simulink model "kalman_estimate_MM"  (R2018b)
settings: Solver=FixedStepAuto  StartTime=0.0  StopTime=500  FixedStep=0.02  RelTol=1e-3
values from neighbouring files (symbols this model uses):
  D = randn(num_output,num_control)    [Com_of_linear_model_calculate.m]    (also in Copy_of_linear_model_calculate.m; D.mat = [0 0 0.00507528406191 0.0236369284061 0.221173094143 0.00198; LINEAR.m = randn(8,1)*10; MM_HKF.m = reshape(out(A_l+B_l+C_l+1:A_l+B_l+C_l+D_l),size_D))
undefined symbols (not defined in the file or in its folder): act_piece, com_piece, piece, sigbuilder_block
libraries: sharedschedule x467, dspsigattribs x44, commchan3 x1
(part 5 of 5)

== system kalman_estimate_MM/sen2_PIECE kalman2/kalman filter1 ==
  A : Inport
  B : Inport  Port=2
  C : Inport  Port=3
  D : Inport  Port=4
  K : Inport  Port=5
  x0 : Inport  Port=6
  Y : Inport  Port=7
  U : Inport  Port=8
  Xtrim : Inport  Port=9
  "\tCX" : Product  Multiplication=Matrix(*)
  AX : Product  Multiplication=Matrix(*)
  BU : Product  Multiplication=Matrix(*)
  Convert 1-D to 2-D1 : dspsigattribs/Convert 1-D to 2-D  M=2  N=1  frameBasedOut=off
      settings: SourceProductName=DSP System Toolbox  SourceProductBaseCode=DS
  DU : Product  Multiplication=Matrix(*)
  Delay : Delay  DelayLength=1  InitialConditionSource=Input port
      settings: InputPortMap=u0,p4
  KY : Product  Multiplication=Matrix(*)
  MATLAB Function : MATLAB Function  TreatAsAtomicUnit=on
  Minus : Sum  Inputs=+-
  Minus1 : Sum
  Minus2 : Sum  Inputs=+-
  Minus3 : Sum  Inputs=+++
  Minus4 : Sum
  X_es : Outport
  Y_es : Outport  Port=2
  Y_error : Outport  Port=3
  wires:
  MATLAB Function/1(y) -> KY/2, Y_error/1
  Minus2/1 -> MATLAB Function/1(u)
  Convert 1-D to 2-D1/1 -> Delay/2
  x0/1 -> Convert 1-D to 2-D1/1
  Minus4/1 -> Minus2/2, Y_es/1
  KY/1 -> Minus3/1
  U/1 -> BU/2, DU/2
  Y/1 -> Minus2/1
  DU/1 -> Minus4/2
  "\tCX"/1 -> Minus4/1
  BU/1 -> Minus3/3
  A/1 -> AX/1
  B/1 -> BU/1
  C/1 -> "\tCX"/1
  D/1 -> DU/1
  K/1 -> KY/1
  Xtrim/1 -> Minus1/2, Minus/2
  Delay/1 -> Minus/1, X_es/1
  Minus/1 -> AX/2, "\tCX"/2
  AX/1 -> Minus3/2
  Minus3/1 -> Minus1/1
  Minus1/1 -> Delay/1

== system kalman_estimate_MM/sen2_PWL/kalman filter1 ==
  A : Inport
  B : Inport  Port=2
  C : Inport  Port=3
  D : Inport  Port=4
  x0 : Inport  Port=5
  U : Inport  Port=6
  Xtrim : Inport  Port=7
  "\tCX" : Product  Multiplication=Matrix(*)
  AX : Product  Multiplication=Matrix(*)
  BU : Product  Multiplication=Matrix(*)
  Convert 1-D to 2-D1 : dspsigattribs/Convert 1-D to 2-D  M=2  N=1  frameBasedOut=off
      settings: SourceProductName=DSP System Toolbox  SourceProductBaseCode=DS
  DU : Product  Multiplication=Matrix(*)
  Delay : Delay  DelayLength=1  InitialConditionSource=Input port
      settings: InputPortMap=u0,p4
  Minus : Sum  Inputs=+-
  Minus1 : Sum
  Minus3 : Sum
  Minus4 : Sum
  X_es : Outport
  Y_es : Outport  Port=2
  wires:
  BU/1 -> Minus3/1
  Convert 1-D to 2-D1/1 -> Delay/2
  x0/1 -> Convert 1-D to 2-D1/1
  Minus4/1 -> Y_es/1
  U/1 -> BU/2, DU/2
  DU/1 -> Minus4/2
  "\tCX"/1 -> Minus4/1
  A/1 -> AX/1
  B/1 -> BU/1
  C/1 -> "\tCX"/1
  D/1 -> DU/1
  Xtrim/1 -> Minus1/2, Minus/2
  Delay/1 -> Minus/1, X_es/1
  Minus/1 -> AX/2, "\tCX"/2
  AX/1 -> Minus3/2
  Minus3/1 -> Minus1/1
  Minus1/1 -> Delay/1

== system kalman_estimate_MM/sen3_PIECE kalman1/kalman filter1 ==
  A : Inport
  B : Inport  Port=2
  C : Inport  Port=3
  D : Inport  Port=4
  K : Inport  Port=5
  x0 : Inport  Port=6
  Y : Inport  Port=7
  U : Inport  Port=8
  Xtrim : Inport  Port=9
  "\tCX" : Product  Multiplication=Matrix(*)
  AX : Product  Multiplication=Matrix(*)
  BU : Product  Multiplication=Matrix(*)
  Convert 1-D to 2-D1 : dspsigattribs/Convert 1-D to 2-D  M=2  N=1  frameBasedOut=off
      settings: SourceProductName=DSP System Toolbox  SourceProductBaseCode=DS
  DU : Product  Multiplication=Matrix(*)
  Delay : Delay  DelayLength=1  InitialConditionSource=Input port
      settings: InputPortMap=u0,p4
  KY : Product  Multiplication=Matrix(*)
  MATLAB Function : MATLAB Function  TreatAsAtomicUnit=on
  Minus : Sum  Inputs=+-
  Minus1 : Sum
  Minus2 : Sum  Inputs=+-
  Minus3 : Sum  Inputs=+++
  Minus4 : Sum
  X_es : Outport
  Y_es : Outport  Port=2
  Y_error : Outport  Port=3
  wires:
  Minus1/1 -> Delay/1
  Minus3/1 -> Minus1/1
  AX/1 -> Minus3/2
  Minus/1 -> "\tCX"/2, AX/2
  Delay/1 -> X_es/1, Minus/1
  Xtrim/1 -> Minus/2, Minus1/2
  K/1 -> KY/1
  D/1 -> DU/1
  C/1 -> "\tCX"/1
  B/1 -> BU/1
  A/1 -> AX/1
  BU/1 -> Minus3/3
  "\tCX"/1 -> Minus4/1
  DU/1 -> Minus4/2
  Y/1 -> Minus2/1
  U/1 -> DU/2, BU/2
  KY/1 -> Minus3/1
  Minus4/1 -> Y_es/1, Minus2/2
  x0/1 -> Convert 1-D to 2-D1/1
  Convert 1-D to 2-D1/1 -> Delay/2
  Minus2/1 -> MATLAB Function/1(u)
  MATLAB Function/1(y) -> Y_error/1, KY/2

== system kalman_estimate_MM/sen3_PIECE kalman3/kalman filter1 ==
  A : Inport
  B : Inport  Port=2
  C : Inport  Port=3
  D : Inport  Port=4
  K : Inport  Port=5
  x0 : Inport  Port=6
  Y : Inport  Port=7
  U : Inport  Port=8
  Xtrim : Inport  Port=9
  "\tCX" : Product  Multiplication=Matrix(*)
  AX : Product  Multiplication=Matrix(*)
  BU : Product  Multiplication=Matrix(*)
  Convert 1-D to 2-D1 : dspsigattribs/Convert 1-D to 2-D  M=2  N=1  frameBasedOut=off
      settings: SourceProductName=DSP System Toolbox  SourceProductBaseCode=DS
  DU : Product  Multiplication=Matrix(*)
  Delay : Delay  DelayLength=1  InitialConditionSource=Input port
      settings: InputPortMap=u0,p4
  KY : Product  Multiplication=Matrix(*)
  MATLAB Function : MATLAB Function  TreatAsAtomicUnit=on
  Minus : Sum  Inputs=+-
  Minus1 : Sum
  Minus2 : Sum  Inputs=+-
  Minus3 : Sum  Inputs=+++
  Minus4 : Sum
  X_es : Outport
  Y_es : Outport  Port=2
  Y_error : Outport  Port=3
  wires:
  MATLAB Function/1(y) -> KY/2, Y_error/1
  Minus2/1 -> MATLAB Function/1(u)
  Convert 1-D to 2-D1/1 -> Delay/2
  x0/1 -> Convert 1-D to 2-D1/1
  Minus4/1 -> Minus2/2, Y_es/1
  KY/1 -> Minus3/1
  U/1 -> BU/2, DU/2
  Y/1 -> Minus2/1
  DU/1 -> Minus4/2
  "\tCX"/1 -> Minus4/1
  BU/1 -> Minus3/3
  A/1 -> AX/1
  B/1 -> BU/1
  C/1 -> "\tCX"/1
  D/1 -> DU/1
  K/1 -> KY/1
  Xtrim/1 -> Minus1/2, Minus/2
  Delay/1 -> Minus/1, X_es/1
  Minus/1 -> AX/2, "\tCX"/2
  AX/1 -> Minus3/2
  Minus3/1 -> Minus1/1
  Minus1/1 -> Delay/1

== system kalman_estimate_MM/sen3_PWL/kalman filter1 ==
  A : Inport
  B : Inport  Port=2
  C : Inport  Port=3
  D : Inport  Port=4
  x0 : Inport  Port=5
  U : Inport  Port=6
  Xtrim : Inport  Port=7
  "\tCX" : Product  Multiplication=Matrix(*)
  AX : Product  Multiplication=Matrix(*)
  BU : Product  Multiplication=Matrix(*)
  Convert 1-D to 2-D1 : dspsigattribs/Convert 1-D to 2-D  M=2  N=1  frameBasedOut=off
      settings: SourceProductName=DSP System Toolbox  SourceProductBaseCode=DS
  DU : Product  Multiplication=Matrix(*)
  Delay : Delay  DelayLength=1  InitialConditionSource=Input port
      settings: InputPortMap=u0,p4
  Minus : Sum  Inputs=+-
  Minus1 : Sum
  Minus3 : Sum
  Minus4 : Sum
  X_es : Outport
  Y_es : Outport  Port=2
  wires:
  BU/1 -> Minus3/1
  Convert 1-D to 2-D1/1 -> Delay/2
  x0/1 -> Convert 1-D to 2-D1/1
  Minus4/1 -> Y_es/1
  U/1 -> BU/2, DU/2
  DU/1 -> Minus4/2
  "\tCX"/1 -> Minus4/1
  A/1 -> AX/1
  B/1 -> BU/1
  C/1 -> "\tCX"/1
  D/1 -> DU/1
  Xtrim/1 -> Minus1/2, Minus/2
  Delay/1 -> Minus/1, X_es/1
  Minus/1 -> AX/2, "\tCX"/2
  AX/1 -> Minus3/2
  Minus3/1 -> Minus1/1
  Minus1/1 -> Delay/1

== system kalman_estimate_MM/sen3_PWL-model/kalman filter1 ==
  A : Inport
  B : Inport  Port=2
  C : Inport  Port=3
  D : Inport  Port=4
  x0 : Inport  Port=5
  U : Inport  Port=6
  Xtrim : Inport  Port=7
  "\tCX" : Product  Multiplication=Matrix(*)
  AX : Product  Multiplication=Matrix(*)
  BU : Product  Multiplication=Matrix(*)
  Convert 1-D to 2-D1 : dspsigattribs/Convert 1-D to 2-D  M=2  N=1  frameBasedOut=off
      settings: SourceProductName=DSP System Toolbox  SourceProductBaseCode=DS
  DU : Product  Multiplication=Matrix(*)
  Delay : Delay  DelayLength=1  InitialConditionSource=Input port
      settings: InputPortMap=u0,p4
  Minus : Sum  Inputs=+-
  Minus1 : Sum
  Minus3 : Sum
  Minus4 : Sum
  X_es : Outport
  Y_es : Outport  Port=2
  wires:
  BU/1 -> Minus3/1
  Convert 1-D to 2-D1/1 -> Delay/2
  x0/1 -> Convert 1-D to 2-D1/1
  Minus4/1 -> Y_es/1
  U/1 -> BU/2, DU/2
  DU/1 -> Minus4/2
  "\tCX"/1 -> Minus4/1
  A/1 -> AX/1
  B/1 -> BU/1
  C/1 -> "\tCX"/1
  D/1 -> DU/1
  Xtrim/1 -> Minus1/2, Minus/2
  Delay/1 -> Minus/1, X_es/1
  Minus/1 -> AX/2, "\tCX"/2
  AX/1 -> Minus3/2
  Minus3/1 -> Minus1/1
  Minus1/1 -> Delay/1

== system kalman_estimate_MM/sen8_PIECE kalman/kalman filter1 ==
  A : Inport
  B : Inport  Port=2
  C : Inport  Port=3
  D : Inport  Port=4
  K : Inport  Port=5
  x0 : Inport  Port=6
  Y : Inport  Port=7
  U : Inport  Port=8
  Xtrim : Inport  Port=9
  "\tCX" : Product  Multiplication=Matrix(*)
  AX : Product  Multiplication=Matrix(*)
  BU : Product  Multiplication=Matrix(*)
  Convert 1-D to 2-D1 : dspsigattribs/Convert 1-D to 2-D  M=2  N=1  frameBasedOut=off
      settings: SourceProductName=DSP System Toolbox  SourceProductBaseCode=DS
  DU : Product  Multiplication=Matrix(*)
  Delay : Delay  DelayLength=1  InitialConditionSource=Input port
      settings: InputPortMap=u0,p4
  KY : Product  Multiplication=Matrix(*)
  MATLAB Function : MATLAB Function  TreatAsAtomicUnit=on
  Minus : Sum  Inputs=+-
  Minus1 : Sum
  Minus2 : Sum  Inputs=+-
  Minus3 : Sum  Inputs=+++
  Minus4 : Sum
  X_es : Outport
  Y_es : Outport  Port=2
  Y_error : Outport  Port=3
  wires:
  MATLAB Function/1(y) -> KY/2, Y_error/1
  Minus2/1 -> MATLAB Function/1(u)
  Convert 1-D to 2-D1/1 -> Delay/2
  x0/1 -> Convert 1-D to 2-D1/1
  Minus4/1 -> Minus2/2, Y_es/1
  KY/1 -> Minus3/1
  U/1 -> BU/2, DU/2
  Y/1 -> Minus2/1
  DU/1 -> Minus4/2
  "\tCX"/1 -> Minus4/1
  BU/1 -> Minus3/3
  A/1 -> AX/1
  B/1 -> BU/1
  C/1 -> "\tCX"/1
  D/1 -> DU/1
  K/1 -> KY/1
  Xtrim/1 -> Minus1/2, Minus/2
  Delay/1 -> Minus/1, X_es/1
  Minus/1 -> AX/2, "\tCX"/2
  AX/1 -> Minus3/2
  Minus3/1 -> Minus1/1
  Minus1/1 -> Delay/1

== system kalman_estimate_MM/sen8_PWL/kalman filter1 ==
  A : Inport
  B : Inport  Port=2
  C : Inport  Port=3
  D : Inport  Port=4
  x0 : Inport  Port=5
  U : Inport  Port=6
  Xtrim : Inport  Port=7
  "\tCX" : Product  Multiplication=Matrix(*)
  AX : Product  Multiplication=Matrix(*)
  BU : Product  Multiplication=Matrix(*)
  Convert 1-D to 2-D1 : dspsigattribs/Convert 1-D to 2-D  M=2  N=1  frameBasedOut=off
      settings: SourceProductName=DSP System Toolbox  SourceProductBaseCode=DS
  DU : Product  Multiplication=Matrix(*)
  Delay : Delay  DelayLength=1  InitialConditionSource=Input port
      settings: InputPortMap=u0,p4
  Minus : Sum  Inputs=+-
  Minus1 : Sum
  Minus3 : Sum
  Minus4 : Sum
  X_es : Outport
  Y_es : Outport  Port=2
  wires:
  BU/1 -> Minus3/1
  Convert 1-D to 2-D1/1 -> Delay/2
  x0/1 -> Convert 1-D to 2-D1/1
  Minus4/1 -> Y_es/1
  U/1 -> BU/2, DU/2
  DU/1 -> Minus4/2
  "\tCX"/1 -> Minus4/1
  A/1 -> AX/1
  B/1 -> BU/1
  C/1 -> "\tCX"/1
  D/1 -> DU/1
  Xtrim/1 -> Minus1/2, Minus/2
  Delay/1 -> Minus/1, X_es/1
  Minus/1 -> AX/2, "\tCX"/2
  AX/1 -> Minus3/2
  Minus3/1 -> Minus1/1
  Minus1/1 -> Delay/1

== matlab function kalman_estimate_MM/data_pre ==
  data: x output; row_data input; y output; y_index input; HP_index input; U_index input; x_index input; U output; HP output; Nx input; Ny input; Nu input
function[x,y,U,HP] = fcn(row_data,y_index,HP_index,U_index,x_index,Nx,Ny,Nu)
%%% 数据相似归一化
% if size(mean_design,1) > size(mean_design,2)
%     mean_ = mean_design';
% else
%     mean_ = mean_design;
% end
if size(y_index,1) > size(y_index,2)
    y_index_ = y_index';
else
    y_index_ =y_index;
end
if size(x_index,1) > size(x_index,2)
    x_index_ = x_index';
else
    x_index_ = x_index;   
end
if size(HP_index,1) > size(HP_index,2)
    HP_index_ = HP_index';
else
    HP_index_ = HP_index;
end
if size(U_index,1) > size(U_index,2)
    U_index_ = U_index';
else
    U_index_ = U_index;
end

if size(row_data,1)>size(row_data,2)
    row = row_data';
else
    row = row_data;
end

y = Ny\row(:,y_index_)';
x = Nx\row(:,x_index_)';
HP = row(:,HP_index_)'-1;
U = Nu\row(:,U_index_)';

== matlab function kalman_estimate_MM/data_pre3 ==
  data: x output; row_data input; y output; y_index input; HP_index input; U_index input; x_index input; U output; HP output; Nx input; Ny input; Nu input
function[x,y,U,HP] = fcn(row_data,y_index,HP_index,U_index,x_index,Nx,Ny,Nu)
%%% 数据相似归一化
% if size(mean_design,1) > size(mean_design,2)
%     mean_ = mean_design';
% else
%     mean_ = mean_design;
% end
if size(y_index,1) > size(y_index,2)
    y_index_ = y_index';
else
    y_index_ =y_index;
end
if size(x_index,1) > size(x_index,2)
    x_index_ = x_index';
else
    x_index_ = x_index;   
end
if size(HP_index,1) > size(HP_index,2)
    HP_index_ = HP_index';
else
    HP_index_ = HP_index;
end
if size(U_index,1) > size(U_index,2)
    U_index_ = U_index';
else
    U_index_ = U_index;
end

if size(row_data,1)>size(row_data,2)
    row = row_data';
else
    row = row_data;
end

y = Ny\row(:,y_index_)';
x = Nx\row(:,x_index_)';
HP = row(:,HP_index_)'-1;
U = Nu\row(:,U_index_)';

== matlab function kalman_estimate_MM/data_pre1 ==
  data: x output; row_data input; y output; y_index input; HP_index input; U_index input; x_index input; U output; HP output
function[x,y,U,HP] = fcn(row_data,y_index,HP_index,U_index,x_index)
%%% 数据相似归一化
% if size(mean_design,1) > size(mean_design,2)
%     mean_ = mean_design';
% else
%     mean_ = mean_design;
% end
if size(y_index,1) > size(y_index,2)
    y_index_ = y_index';
else
    y_index_ =y_index;
end
if size(x_index,1) > size(x_index,2)
    x_index_ = x_index';
else
    x_index_ = x_index;   
end
if size(HP_index,1) > size(HP_index,2)
    HP_index_ = HP_index';
else
    HP_index_ = HP_index;
end
if size(U_index,1) > size(U_index,2)
    U_index_ = U_index';
else
    U_index_ = U_index;
end

if size(row_data,1)>size(row_data,2)
    row = row_data';
else
    row = row_data;
end

y = row(:,y_index_)';
x = row(:,x_index_)';
HP = row(:,HP_index_)'-1;
U = row(:,U_index_)';

== matlab function kalman_estimate_MM/PIECE kalman/kalman filter1/MATLAB Function ==
  data: u input; y output
function y = fcn(u)
u(1) = 0;
y = u;

== matlab function kalman_estimate_MM/HKF1/kalman filter1/MATLAB Function ==
  data: u input; y output
function y = fcn(u)
u(1) = 0;
y = u;

== matlab function kalman_estimate_MM/HKF3/kalman filter1/MATLAB Function ==
  data: u input; y output
function y = fcn(u)
u(1) = 0;
y = u;

== matlab function kalman_estimate_MM/HKF4/kalman filter1/MATLAB Function ==
  data: u input; y output
function y = fcn(u)
u(1) = 0;
y = u;

== matlab function kalman_estimate_MM/real_engine ==
  data: x output; row_data input; y output; y_index input; HP_index input; U_index input; x_index input; U output; HP output; Nx input; Ny input; Nu input
function[x,y,U,HP] = fcn(row_data,y_index,HP_index,U_index,x_index,Nx,Ny,Nu)
%%% 数据相似归一化
% if size(mean_design,1) > size(mean_design,2)
%     mean_ = mean_design';
% else
%     mean_ = mean_design;
% end
if size(y_index,1) > size(y_index,2)
    y_index_ = y_index';
else
    y_index_ =y_index;
end
if size(x_index,1) > size(x_index,2)
    x_index_ = x_index';
else
    x_index_ = x_index;   
end
if size(HP_index,1) > size(HP_index,2)
    HP_index_ = HP_index';
else
    HP_index_ = HP_index;
end
if size(U_index,1) > size(U_index,2)
    U_index_ = U_index';
else
    U_index_ = U_index;
end

if size(row_data,1)>size(row_data,2)
    row = row_data';
else
    row = row_data;
end

y = Ny\row(:,y_index_)';
x = Nx\row(:,x_index_)';
HP = row(:,HP_index_)'-1;
U = Nu\row(:,U_index_)';

== matlab function kalman_estimate_MM/health_PWL/MATLAB Function ==
  data: err input; y output; S input
function y = fcn(err,S)
y = exp(-0.5*err'*inv(S)*err);
end

== matlab function kalman_estimate_MM/MATLAB Function3 ==
  data: mag input; y output; no input; y_design input
function y = fcn(mag,no,y_design)
y_ = zeros(1,10);
y_(no) = mag;
y = y_';
end

== matlab function kalman_estimate_MM/MATLAB Function4 ==
  data: mag input; y output; no input; y_design input
function y = fcn(mag,no,y_design)
y_ = zeros(1,10);
y_(no) = mag;
y = y_';
end

== matlab function kalman_estimate_MM/MATLAB Function5 ==
  data: mag input; y output; no input; y_design input
function y = fcn(mag,no,y_design)
y_ = zeros(1,10);
y_(no) = mag;
y = y_';
end

== matlab function kalman_estimate_MM/PIECE kalman1/kalman filter1/MATLAB Function ==
  data: u input; y output
function y = fcn(u)
u(1) = 0;
y = u;

== matlab function kalman_estimate_MM/MATLAB Function ==
  data: mag input; y output; no input; y_design input
function y = fcn(mag,no,y_design)
y_ = zeros(1,10);
y_(no) = mag;
y = y_';
end

== matlab function kalman_estimate_MM/sen2_PIECE kalman2/kalman filter1/MATLAB Function ==
  data: u input; y output
function y = fcn(u)
u(1) = 0;
y = u;

== matlab function kalman_estimate_MM/HKF5/kalman filter1/MATLAB Function ==
  data: u input; y output
function y = fcn(u)
u(1) = 0;
y = u;

== matlab function kalman_estimate_MM/HKF6/kalman filter1/MATLAB Function ==
  data: u input; y output
function y = fcn(u)
u(1) = 0;
y = u;

== matlab function kalman_estimate_MM/HKF7/kalman filter1/MATLAB Function ==
  data: u input; y output
function y = fcn(u)
u(1) = 0;
y = u;

== matlab function kalman_estimate_MM/sen3_PIECE kalman3/kalman filter1/MATLAB Function ==
  data: u input; y output
function y = fcn(u)
u(1) = 0;
y = u;

== matlab function kalman_estimate_MM/HKF3/MATLAB Function ==
  data: err input; y output; S input
function y = fcn(err,S)
y = exp(-0.5*err'*inv(S)*err);
end

== matlab function kalman_estimate_MM/HKF4/MATLAB Function ==
  data: err input; y output; S input
function y = fcn(err,S)
y = exp(-0.5*err'*inv(S)*err);
end

== matlab function kalman_estimate_MM/HKF1/MATLAB Function ==
  data: err input; y output; S input
function y = fcn(err,S)
y = exp(-0.5*err'*inv(S)*err);
end

== matlab function kalman_estimate_MM/sen8_PIECE kalman/kalman filter1/MATLAB Function ==
  data: u input; y output
function y = fcn(u)
u(1) = 0;
y = u;

== matlab function kalman_estimate_MM/HKF5/MATLAB Function ==
  data: err input; y output; S input
function y = fcn(err,S)
y = exp(-0.5*err'*inv(S)*err);
end

== matlab function kalman_estimate_MM/HKF6/MATLAB Function ==
  data: err input; y output; S input
function y = fcn(err,S)
y = exp(-0.5*err'*inv(S)*err);
end

== matlab function kalman_estimate_MM/HKF7/MATLAB Function ==
  data: err input; y output; S input
function y = fcn(err,S)
y = exp(-0.5*err'*inv(S)*err);
end

== matlab function kalman_estimate_MM/MATLAB Function8 ==
  data: u input; y output; p0 input
function y = fcn(u,p0)
%#codegen
u_ = reshape(u,[1,length(u)]);
p0_ = reshape(p0,[1,length(p0)]);
u_sum = u_*p0_';
y = u_.*p0_./u_sum;
y(y <0.00001) = 0.00001;
% if max(y)<=0.99
%     y(1:end-1) = 0;
%     y(end) = 1;
% end
end

== matlab function kalman_estimate_MM/data_pre2 ==
  data: x output; row_data input; y output; y_index input; HP_index input; U_index input; x_index input; U output; HP output; Nx input; Ny input; Nu input
function[x,y,U,HP] = fcn(row_data,y_index,HP_index,U_index,x_index,Nx,Ny,Nu)
%%% 数据相似归一化
% if size(mean_design,1) > size(mean_design,2)
%     mean_ = mean_design';
% else
%     mean_ = mean_design;
% end
if size(y_index,1) > size(y_index,2)
    y_index_ = y_index';
else
    y_index_ =y_index;
end
if size(x_index,1) > size(x_index,2)
    x_index_ = x_index';
else
    x_index_ = x_index;   
end
if size(HP_index,1) > size(HP_index,2)
    HP_index_ = HP_index';
else
    HP_index_ = HP_index;
end
if size(U_index,1) > size(U_index,2)
    U_index_ = U_index';
else
    U_index_ = U_index;
end

if size(row_data,1)>size(row_data,2)
    row = row_data';
else
    row = row_data;
end

y = Ny\row(:,y_index_)';
x = Nx\row(:,x_index_)';
HP = row(:,HP_index_)'-1;
U = Nu\row(:,U_index_)';

== matlab function kalman_estimate_MM/HKF9/MATLAB Function ==
  data: err input; y output; S input
function y = fcn(err,S)
y = exp(-0.5*err'*inv(S)*err);
end

== matlab function kalman_estimate_MM/HKF9/kalman filter1/MATLAB Function ==
  data: u input; y output
function y = fcn(u)
u(1) = 0;
y = u;

== matlab function kalman_estimate_MM/com_PIECE kalman/kalman filter1/MATLAB Function ==
  data: u input; y output
function y = fcn(u)
u(1) = 0;
y = u;

== matlab function kalman_estimate_MM/act_PIECE kalman/kalman filter1/MATLAB Function ==
  data: u input; y output
function y = fcn(u)
u(1) = 0;
y = u;

== matlab function kalman_estimate_MM/PIECE kalman1/MATLAB Function ==
  data: err input; y output; S input
function y = fcn(err,S)
y = exp(-0.5*err'*inv(S)*err);
end

== matlab function kalman_estimate_MM/sen2_PIECE kalman2/MATLAB Function ==
  data: err input; y output; S input
function y = fcn(err,S)
y = exp(-0.5*err'*inv(S)*err);
end

== matlab function kalman_estimate_MM/sen3_PIECE kalman3/MATLAB Function ==
  data: err input; y output; S input
function y = fcn(err,S)
y = exp(-0.5*err'*inv(S)*err);
end

== matlab function kalman_estimate_MM/sen8_PIECE kalman/MATLAB Function ==
  data: err input; y output; S input
function y = fcn(err,S)
y = exp(-0.5*err'*inv(S)*err);
end

== matlab function kalman_estimate_MM/com_PIECE kalman/MATLAB Function ==
  data: err input; y output; S input
function y = fcn(err,S)
y = exp(-0.5*err'*inv(S)*err);
end

== matlab function kalman_estimate_MM/act_PIECE kalman/MATLAB Function ==
  data: err input; y output; S input
function y = fcn(err,S)
y = exp(-0.5*err'*inv(S)*err);
end

== matlab function kalman_estimate_MM/MATLAB Function1 ==
  data: u input; y output; p0 input
function y = fcn(u,p0)
%#codegen
u_ = reshape(u,[1,length(u)]);
p0_ = reshape(p0,[1,length(p0)]);
u_sum = u_*p0_';
y = u_.*p0_./u_sum;
y(y <0.00001) = 0.00001;
% if max(y)<=0.99
%     y(1:end-1) = 0;
%     y(end) = 1;
% end
end

== matlab function kalman_estimate_MM/sen3_PIECE kalman1/MATLAB Function ==
  data: err input; y output; S input
function y = fcn(err,S)
y = exp(-0.5*err'*inv(S)*err);
end

== matlab function kalman_estimate_MM/sen3_PIECE kalman1/kalman filter1/MATLAB Function ==
  data: u input; y output
function y = fcn(u)
u(1) = 0;
y = u;

== matlab function kalman_estimate_MM/MATLAB Function2 ==
  data: mag input; y output; no input; y_design input
function y = fcn(mag,no,y_design)
y_ = zeros(1,10);
y_(no) = mag;
y = y_';
end
